simulink model "PID_Controller"  (R2015a)
settings: Solver=FixedStepDiscrete  StartTime=0.0  StopTime=10.0  FixedStep=delta_t  RelTol=1e-3
undefined symbols (not defined in the file): D, delta_t, I, Kd, Kp, M_tilde, psi_dot_max, psi_max, S, S_pinv
settings Model: Creator=Kerianne  LastModifiedBy=Kerianne
settings DataIOCC: SaveFormat=Structure
settings OptimizationCC: InlineParams=on  ExpressionDepthLimit=2147483647
settings DebuggingCC: UnderspecifiedInitializationDetection=Classic  MergeDetectMultiDrivingBlocksExec=none  SolverPrmCheckMsg=warning  StateNameClashWarn=warning

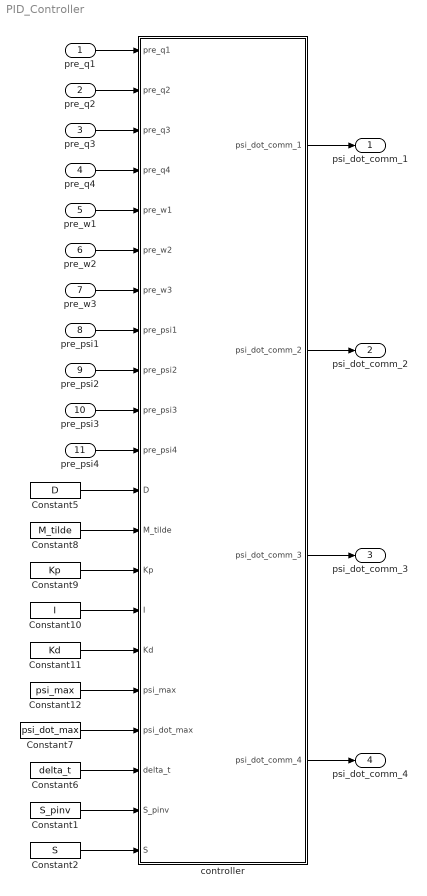
== system PID_Controller ==
  pre_q1 : Inport
  pre_q2 : Inport  Port=2
  pre_q3 : Inport  Port=3
  pre_q4 : Inport  Port=4
  pre_w1 : Inport  Port=5
  pre_w2 : Inport  Port=6
  pre_w3 : Inport  Port=7
  pre_psi1 : Inport  Port=8
  pre_psi2 : Inport  Port=9
  pre_psi3 : Inport  Port=10
  pre_psi4 : Inport  Port=11
  Constant1 : Constant  Value=S_pinv
  Constant10 : Constant  Value=I
  Constant11 : Constant  Value=Kd
  Constant12 : Constant  Value=psi_max
  Constant2 : Constant  Value=S
  Constant5 : Constant  Value=D
  Constant6 : Constant  Value=delta_t
  Constant7 : Constant  Value=psi_dot_max
  Constant8 : Constant  Value=M_tilde
  Constant9 : Constant  Value=Kp
  controller : MATLAB Function  TreatAsAtomicUnit=on
  psi_dot_comm_1 : Outport
  psi_dot_comm_2 : Outport  Port=2
  psi_dot_comm_3 : Outport  Port=3
  psi_dot_comm_4 : Outport  Port=4
  wires:
  Constant6/1 -> controller/19(delta_t)
  Constant7/1 -> controller/18(psi_dot_max)
  Constant12/1 -> controller/17(psi_max)
  Constant11/1 -> controller/16(Kd)
  Constant10/1 -> controller/15(I)
  Constant9/1 -> controller/14(Kp)
  Constant8/1 -> controller/13(M_tilde)
  Constant5/1 -> controller/12(D)
  pre_psi3/1 -> controller/10(pre_psi3)
  pre_psi2/1 -> controller/9(pre_psi2)
  pre_psi1/1 -> controller/8(pre_psi1)
  pre_w3/1 -> controller/7(pre_w3)
  pre_w2/1 -> controller/6(pre_w2)
  pre_w1/1 -> controller/5(pre_w1)
  pre_q4/1 -> controller/4(pre_q4)
  pre_q3/1 -> controller/3(pre_q3)
  pre_q2/1 -> controller/2(pre_q2)
  pre_q1/1 -> controller/1(pre_q1)
  controller/3(psi_dot_comm_3) -> psi_dot_comm_3/1
  controller/1(psi_dot_comm_1) -> psi_dot_comm_1/1
  controller/2(psi_dot_comm_2) -> psi_dot_comm_2/1
  Constant1/1 -> controller/20(S_pinv)
  controller/4(psi_dot_comm_4) -> psi_dot_comm_4/1
  pre_psi4/1 -> controller/11(pre_psi4)
  Constant2/1 -> controller/21(S)

== matlab function PID_Controller/controller ==
  data: pre_q1 input; pre_q2 input; pre_q3 input; pre_q4 input; pre_w1 input; pre_w2 input; pre_w3 input; pre_psi1 input; pre_psi2 input; pre_psi3 input; pre_psi4 input; psi_dot_comm_1 output; D input; M_tilde input; Kp input; I input; Kd input; psi_max input; psi_dot_max input; delta_t input; psi_dot_comm_2 output; psi_dot_comm_3 output; psi_dot_comm_4 output; S_pinv input; S input
function [psi_dot_comm_1, psi_dot_comm_2, psi_dot_comm_3,psi_dot_comm_4] = fcn(pre_q1,pre_q2,pre_q3,pre_q4,pre_w1,pre_w2,pre_w3,pre_psi1,pre_psi2,pre_psi3,pre_psi4,D,M_tilde,Kp,I,Kd,psi_max,psi_dot_max,delta_t,S_pinv,S)
% 14 Aug 2015
% States at the end fot he last time step
    q       = [pre_q1,pre_q2,pre_q3,pre_q4];    %s/c quaternion
    omega   = [pre_w1,pre_w2,pre_w3];           %s/c angular rates 
    psi     = [pre_psi1,pre_psi2,pre_psi3,pre_psi4];     %RWA angle rates
    
    % Compute reaction wheel array angular momentum
    h_rwa = S*psi';
    
    % Error between current quaternion and desired final quaternion
    q_error = M_tilde*q';
    
    % Computed control
    h_dot_rwa = Kp*I*q_error(1:3,1)+Kd*I*omega'-skew(omega')*(I*omega'+h_rwa);
    psi_dot = S_pinv*h_dot_rwa;
    psi_dot_comm_1 = psi_dot(1);
    psi_dot_comm_2 = psi_dot(2);
    psi_dot_comm_3 = psi_dot(3);
    psi_dot_comm_4 = psi_dot(4);
    
    % Check that commanded psi_dot does not exceed max_psi_dot limitation
    % of the RW, and if it does, set to the max
    if abs(psi_dot_comm_1) >= psi_dot_max
        psi_dot_comm_1 = sign(psi_dot_comm_1)*psi_dot_max;
    end
    if abs(psi_dot_comm_2) >= psi_dot_max
        psi_dot_comm_2 = sign(psi_dot_comm_2)*psi_dot_max;
    end
    if abs(psi_dot_comm_3) >= psi_dot_max
        psi_dot_comm_3 = sign(psi_dot_comm_3)*psi_dot_max;
    end
    if abs(psi_dot_comm_4) >= psi_dot_max
        psi_dot_comm_4 = sign(psi_dot_comm_4)*psi_dot_max;
    end
    % Check if the commanded psi_dot would exceed max psi limitation, if so
    % set the commanded psi_dot to 0
    if abs(psi(1)+ psi_dot_comm_1*delta_t) >= psi_max
        psi_dot_comm_1 = 0;
    end
    if abs(psi(2)+ psi_dot_comm_2*delta_t) >= psi_max
        psi_dot_comm_2 = 0;
    end
    if abs(psi(3)+ psi_dot_comm_3*delta_t) >= psi_max
        psi_dot_comm_3 = 0;
    end
    if abs(psi(4)+ psi_dot_comm_4*delta_t) >= psi_max
        psi_dot_comm_4 = 0;
    end
